simulink model "Ques3_system"  (R2020b)
settings: Solver=VariableStepAuto  StartTime=0.0  StopTime=10.0  RelTol=1e-3
settings Model: Creator=sneha  LastModifiedBy=sneha

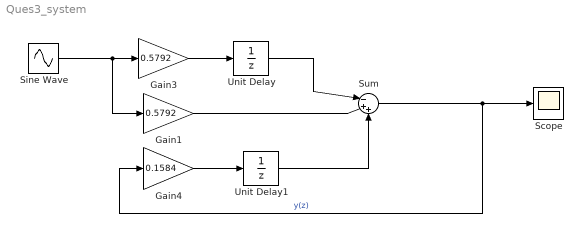
== system Ques3_system ==
  Gain1 : Gain  Gain=0.5792
  Gain3 : Gain  Gain=0.5792
  Gain4 : Gain  Gain=0.1584
  Scope : Scope
  Sine Wave : Sin  SampleTime=0
  Sum : Sum  Inputs=|-++
  Unit Delay : UnitDelay  SampleTime=-1  HasFrameUpgradeWarning=on
  Unit Delay1 : UnitDelay  SampleTime=-1  HasFrameUpgradeWarning=on
  wires:
  Gain1/1 -> Sum/2
  Gain3/1 -> Unit Delay/1
  Sine Wave/1 -> Gain1/1, Gain3/1
  Sum/1 -> Scope/1, Gain4/1  "y(z)"
  Unit Delay/1 -> Sum/1
  Gain4/1 -> Unit Delay1/1
  Unit Delay1/1 -> Sum/3
